simulink library "lib_road"  (R2026a)
settings: Solver=VariableStepAuto
settings Model: Creator=alessandro-nardin  LastModifiedBy=alessandro-nardin

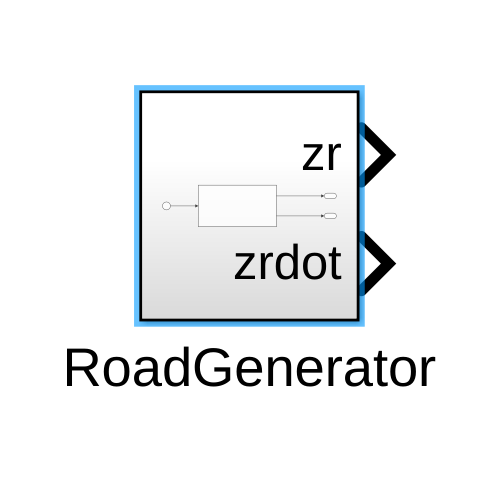
[thumbnail: Simulink's stored preview of the top-level diagram]
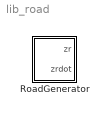
== system lib_road ==
  RoadGenerator : Subsystem

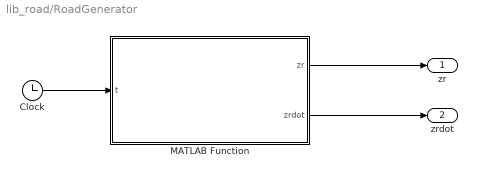
== system lib_road/RoadGenerator ==
  Clock : Clock
  MATLAB Function : MATLAB Function  TreatAsAtomicUnit=on
  zr : Outport
  zrdot : Outport  Port=2
  wires:
  Clock/1 -> MATLAB Function/1(t)
  MATLAB Function/1(zr) -> zr/1
  MATLAB Function/2(zrdot) -> zrdot/1

== matlab function lib_road/RoadGenerator/MATLAB Function ==
  data: t input; zr output; zrdot output; road_param parameter
function [zr, zrdot] = road_generation(t, road_param)
    zr    = road_gen(t, road_param);
    zrdot = road_dot_gen(t, road_param);
end
